simulink model "simulate_QAM_fixed_partial"  (R2021a)
settings: Solver=VariableStepAuto  StartTime=0.0  StopTime=1  RelTol=1e-3
InitFcn:
  | fs = 4000;
  | frameSize = 512;
libraries: dspsrcs4 x4
settings Model: Creator=Byung-Jun Jang  LastModifiedBy=user
settings SolverCC: AlgebraicLoopSolver=TrustRegion
settings DataIOCC: ReturnWorkspaceOutputs=off
settings DebuggingCC: SFMachineParentedDataDiag=warning  ArithmeticOperatorsInVariantConditions=warning
settings SFSimCC: SimUseLocalCustomCode=off  CustomCodeUndefinedFunction=UseInterfaceOnly
settings RTWCC: RTWUseLocalCustomCode=off
settings CodeAppCC: StateflowObjectComments=on
settings SimscapeCC: SimscapeNormalizeSystem=off

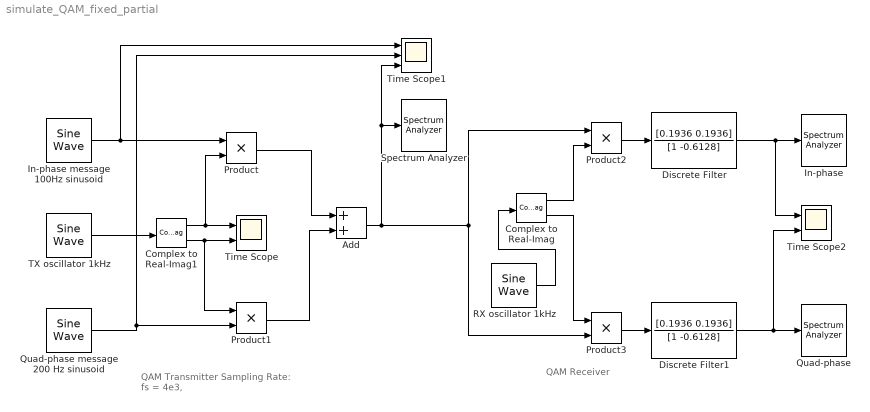
== system simulate_QAM_fixed_partial ==
  note: QAM Transmitter
      | Sampling Rate: fs = 4e3,
  note: QAM Receiver
  Add : Sum  OutDataTypeStr=T8  RndMeth=Nearest  SaturateOnIntegerOverflow=on
  Complex to Real-Imag : ComplexToRealImag
  Complex to Real-Imag1 : ComplexToRealImag
  Discrete Filter : DiscreteFilter  Numerator=[0.1936 0.1936]  Denominator=[1 -0.6128]  InputProcessing=Columns as channels (frame based)  FilterStructure=Direct form II transposed  a0EqualsOne=on  StateDataTypeStr=T8  NumCoefDataTypeStr=T8  DenCoefDataTypeStr=T8  NumProductDataTypeStr=T8  DenProductDataTypeStr=T8  NumAccumDataTypeStr=T8  DenAccumDataTypeStr=T8  OutDataTypeStr=T8  RndMeth=Nearest  SaturateOnIntegerOverflow=on
  Discrete Filter1 : DiscreteFilter  Numerator=[0.1936 0.1936]  Denominator=[1 -0.6128]  InputProcessing=Columns as channels (frame based)  FilterStructure=Direct form II transposed  a0EqualsOne=on  StateDataTypeStr=T8  NumCoefDataTypeStr=T8  DenCoefDataTypeStr=T8  NumProductDataTypeStr=T8  DenProductDataTypeStr=T8  NumAccumDataTypeStr=T8  DenAccumDataTypeStr=T8  OutDataTypeStr=T8  RndMeth=Nearest  SaturateOnIntegerOverflow=on
  In-phase : SpectrumAnalyzer
  In-phase message 100Hz sinusoid : dspsrcs4/Sine Wave  Amplitude=1  Frequency=100  Phase=90  SampleMode=Discrete  OutComplex=Real  CompMethod=Trigonometric fcn  TableSize=Speed  SampleTime=1/fs  SamplesPerFrame=frameSize  ResetState=Restart at time zero  OutputFrames=off  dataType=double  wordLen=16  udDataType=sfix(16)  fracBitsMode=Best precision  numFracBits=15  OutDataTypeStr=double  LastOutDataTypeStr=double
  Product{,1..3} (4 alike) : Product  OutDataTypeStr=T8  RndMeth=Nearest  SaturateOnIntegerOverflow=on
  Quad-phase : SpectrumAnalyzer
  Quad-phase message 200 Hz sinusoid : dspsrcs4/Sine Wave  Amplitude=1  Frequency=200  Phase=0  SampleMode=Discrete  OutComplex=Real  CompMethod=Trigonometric fcn  TableSize=Speed  SampleTime=1/fs  SamplesPerFrame=frameSize  ResetState=Restart at time zero  OutputFrames=off  dataType=double  wordLen=16  udDataType=sfix(16)  fracBitsMode=Best precision  numFracBits=15  OutDataTypeStr=double  LastOutDataTypeStr=double
  RX oscillator 1kHz : dspsrcs4/Sine Wave  Amplitude=sqrt(2)  Frequency=1000  Phase=0  SampleMode=Discrete  OutComplex=Complex  CompMethod=Trigonometric fcn  TableSize=Speed  SampleTime=1/fs  SamplesPerFrame=frameSize  ResetState=Restart at time zero  OutputFrames=off  dataType=double  wordLen=16  udDataType=sfix(16)  fracBitsMode=Best precision  numFracBits=15  OutDataTypeStr=double  LastOutDataTypeStr=double
  Spectrum Analyzer : SpectrumAnalyzer
  TX oscillator 1kHz : dspsrcs4/Sine Wave  Amplitude=sqrt(2)  Frequency=1000  Phase=0  SampleMode=Discrete  OutComplex=Complex  CompMethod=Trigonometric fcn  TableSize=Speed  SampleTime=1/fs  SamplesPerFrame=frameSize  ResetState=Restart at time zero  OutputFrames=off  dataType=double  wordLen=16  udDataType=sfix(16)  fracBitsMode=Best precision  numFracBits=15  OutDataTypeStr=double  LastOutDataTypeStr=double
  Time Scope : Scope  NumInputPorts=2
  Time Scope1 : Scope  NumInputPorts=3
  Time Scope2 : Scope  NumInputPorts=2
  wires:
  In-phase message 100Hz sinusoid/1 -> Time Scope1/1, Product/1
  Product/1 -> Add/1
  Quad-phase message 200 Hz sinusoid/1 -> Time Scope1/2, Product1/2
  Product1/1 -> Add/2
  Complex to Real-Imag/1 -> Product2/2
  Add/1 -> Product3/2, Product2/1, Spectrum Analyzer/1, Time Scope1/3
  Product3/1 -> Discrete Filter1/1
  Product2/1 -> Discrete Filter/1
  Discrete Filter/1 -> In-phase/1, Time Scope2/1
  Complex to Real-Imag/2 -> Product3/1
  RX oscillator 1kHz/1 -> Complex to Real-Imag/1
  Discrete Filter1/1 -> Time Scope2/2, Quad-phase/1
  Complex to Real-Imag1/2 -> Product1/1, Time Scope/2
  TX oscillator 1kHz/1 -> Complex to Real-Imag1/1
  Complex to Real-Imag1/1 -> Product/2, Time Scope/1
